simulink model "A03_L1_1_extins"  (R2014b)
settings: Solver=ode45  StartTime=0.0  StopTime=8  RelTol=1e-3
libraries: simulink x6
settings Model: Creator=User  LastModifiedBy=User

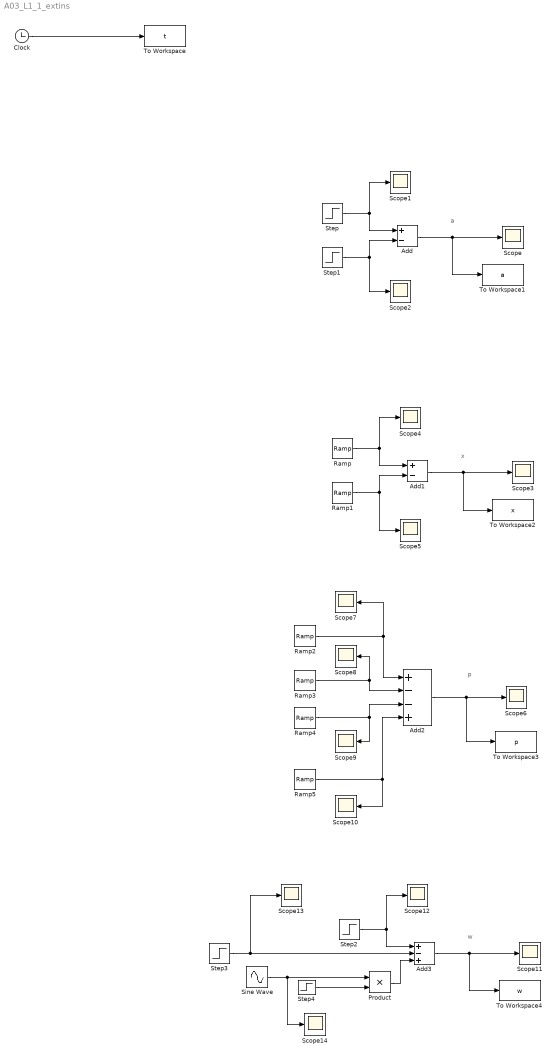
== system A03_L1_1_extins ==
  note: a
  note: x
  note: p
  note: w
  Add : Sum  Inputs=+-
  Add1 : Sum  Inputs=+-
  Add2 : Sum  Inputs=+--+
  Add3 : Sum  Inputs=+-+
  Clock : Clock
  Product : Product
  Ramp : simulink/Sources/Ramp  slope=0.8  start=2  X0=0
  Ramp1 : simulink/Sources/Ramp  slope=0.8  start=3  X0=0
  Ramp2 : simulink/Sources/Ramp  slope=0.8  start=2  X0=0
  Ramp3 : simulink/Sources/Ramp  slope=0.8  start=3  X0=0
  Ramp4 : simulink/Sources/Ramp  slope=0.8  start=6  X0=0
  Ramp5 : simulink/Sources/Ramp  slope=0.8  start=7  X0=0
  Scope{,1..14} (15 alike) : Scope
      Scope settings: TimeRange=5
      Scope1 settings: TimeRange=5
      Scope10 settings: TimeRange=5  SaveName=ScopeData10
      Scope11 settings: TimeRange=5  SaveName=ScopeData11
      Scope12 settings: TimeRange=5  SaveName=ScopeData12
      Scope13 settings: TimeRange=5  SaveName=ScopeData13
      Scope14 settings: TimeRange=5  SaveName=ScopeData14
      Scope2 settings: TimeRange=5  SaveName=ScopeData2
      Scope3 settings: TimeRange=5  SaveName=ScopeData3
      Scope4 settings: TimeRange=5  SaveName=ScopeData4
      Scope5 settings: TimeRange=5  SaveName=ScopeData5
      Scope6 settings: TimeRange=5  SaveName=ScopeData6
      Scope7 settings: TimeRange=5  SaveName=ScopeData7
      Scope8 settings: TimeRange=5  SaveName=ScopeData8
      Scope9 settings: TimeRange=5  SaveName=ScopeData9
  Sine Wave : Sin  Amplitude=0.2  Frequency=7  SampleTime=0
  Step : Step  After=1.5  SampleTime=0
  Step1 : Step  Time=3  After=1.5  SampleTime=0
  Step2 : Step  After=1.5  SampleTime=0
  Step3 : Step  Time=3  After=1.5  SampleTime=0
  Step4 : Step  Time=6  Before=1  After=0  SampleTime=0
  To Workspace : ToWorkspace  VariableName=t  SampleTime=-1
  To Workspace1 : ToWorkspace  VariableName=a  SampleTime=-1
  To Workspace2 : ToWorkspace  VariableName=x  SampleTime=-1
  To Workspace3 : ToWorkspace  VariableName=p  SampleTime=-1
  To Workspace4 : ToWorkspace  VariableName=w  SampleTime=-1
  wires:
  Clock/1 -> To Workspace/1
  Step/1 -> Add/1, Scope1/1
  Step1/1 -> Scope2/1, Add/2
  Add/1 -> To Workspace1/1, Scope/1
  Ramp/1 -> Add1/1, Scope4/1
  Ramp1/1 -> Scope5/1, Add1/2
  Add1/1 -> To Workspace2/1, Scope3/1
  Ramp2/1 -> Add2/1, Scope7/1
  Ramp3/1 -> Add2/2, Scope8/1
  Add2/1 -> Scope6/1, To Workspace3/1
  Ramp4/1 -> Add2/3, Scope9/1
  Ramp5/1 -> Add2/4, Scope10/1
  Step2/1 -> Add3/1, Scope12/1
  Step3/1 -> Scope13/1, Add3/2
  Add3/1 -> To Workspace4/1, Scope11/1
  Product/1 -> Add3/3
  Sine Wave/1 -> Scope14/1, Product/1
  Step4/1 -> Product/2
